simulink model "b0307"  (R2025b)
settings: Solver=ode4  StartTime=0.0  StopTime=533  FixedStep=0.001  RelTol=1e-3
values from neighbouring files (symbols this model uses):
  alpha_vector = [-8 -4 -2 0 2 3 4 5 6 8 10 12]    [aerodata.mat]    (also in airdate.m = [-8 -4 -2 0 2 3 4 5 6 8 10 12]')
  alpha_vector1 = [-4 0 4 8]    [aerodata.mat]    (also in airdate.m = [-4, 0, 4, 8])
  alpha_vector2 = [-4 0 4 8]    [aerodata.mat]    (also in airdate.m = [-4, 0, 4, 8])
  b_ref = 2.24    [init.m]
  beta_vector1 = [-8 -4 0 4 8]    [aerodata.mat]    (also in airdate.m = [-8, -4, 0, 4, 8])
  c_ref = 0.165    [init.m]
  CD_alpha = [0.0485620740363 0.0318356514345 0.0317790643102 0.0364045204537 0.0445214008185 0.0513240541996 0.0580305477533 0.0657045426134 0.0744839493029 0.0955551011208 0.133141813384 0.18014601666]    [aerodata.mat]    (also in airdate.m = alpha_matrix(1:length(alpha_vector), 3))
  CD_beta = [0.0413061898506 0.0345389961433 0.0318356514345 0.0345389961433 0.0413061898506 0.0436826 0.0385768 0.0364045204537 0.0371657170379 0.0408604078007 0.0616785 0.0590205 ... (20 elements, 5x4)]    [aerodata.mat]    (also in airdate.m = reshape(beta_matrix(:, 3), [n_beta, n_alpha1]))
  CD_ELE = [0.0367807192259 0.0308673912055 0.0306770192219 0.0329799710874 0.0376266798938 0.0362372767671 0.0347486720958 0.0364045204537 0.0395900797854 0.0493584368547 0.0520155680915 0.0546030505455 ... (20 elements, 5x4)]    [aerodata.mat]    (also in airdate.m = reshape(def_ELE_L_matrix(:, 4), [n_ele, n_alpha2]))
  CL_alpha = [-0.316928256932 -0.0246785813034 0.130283368141 0.288945629191 0.449323999783 0.525648685194 0.60297649153 0.678148219772 0.750129216407 0.872962476804 0.920788454091 0.929116005788]    [aerodata.mat]    (also in airdate.m = alpha_matrix(1:length(alpha_vector), 5))
  Cl_alpha = [-0.000640872979326 1.08116418077e-05 2.92649499784e-07 0 -0.000437066219056 -0.000762440123061 -0.000973039479867 -0.00125684277681 -0.00152984821199 -0.00187186802219 -0.00184918573213 0.00105936824418]    [aerodata.mat]    (also in airdate.m = alpha_matrix(1:length(alpha_vector), 6))
  CL_beta = [-0.0254603323809 -0.0249297140554 -0.0246785813034 -0.0249297140554 -0.0254603323809 0.27807 0.286078 0.288945629191 0.286671909097 0.27925707766 0.602944 0.604359 ... (20 elements, 5x4)]    [aerodata.mat]    (also in airdate.m = reshape(beta_matrix(:, 5), [n_beta, n_alpha1]))
  Cl_beta = [0.000236297001567 0.000139283426539 1.08116418077e-05 -0.000139283426539 -0.000236297001567 0.000738099 0.000299952 -0.000269027677603 -0.00096883985561 -0.00179948469019 0.0018278 0.000411742 ... (20 elements, 5x4)]    [aerodata.mat]    (also in airdate.m = reshape(beta_matrix(:, 6), [n_beta, n_alpha1]))
  CL_ELE = [-0.209245674304 -0.118097376915 -0.0691301102129 -0.0258480382303 0.0604619193477 0.145712419951 0.241076881119 0.288945629191 0.337037782187 0.427489906586 0.461138992576 0.556875751161 ... (20 elements, 5x4)]    [aerodata.mat]    (also in airdate.m = reshape(def_ELE_L_matrix(:, 6), [n_ele, n_alpha2]))
  Cl_ELE = [-0.0251269797289 -0.008426817179 0.000240167384607 0.00909972758991 0.0243415498089 -0.0265884432031 -0.00914521718395 -0.000269027677603 0.00845228310052 0.0248325485851 -0.027436226674 -0.00980497383292 ... (20 elements, 5x4)]    [aerodata.mat]    (also in airdate.m = reshape(def_ELE_L_matrix(:, 7), [n_ele, n_alpha2]))
  Cl_ELER = [0.0251269797289 0.008426817179 -0.000240167384607 -0.00909972758991 -0.0243415498089 0.0265884432031 0.00914521718395 0.000269027677603 -0.00845228310052 -0.0248325485851 0.027436226674 0.00980497383292 ... (20 elements, 5x4)]    [aerodata.mat]    (also in airdate.m = -Cl_ELE)
  Cm_alpha = [0.0626600725128 0.0530799370217 0.0636683163616 0.0662391704182 0.0712518097577 0.059404297375 0.0463976401398 0.0265816846325 -0.000744425674427 -0.0975303788137 -0.390110677431 -0.549514574144]    [aerodata.mat]    (also in airdate.m = alpha_matrix(1:length(alpha_vector), 7))
  Cm_beta = [0.0443576401398 0.0504624 0.0530799370217 0.0504624 0.0443576401398 0.0399653 0.0540624 0.0662391704182 0.0664956832735 0.054831924477 -0.0180401 0.0135503 ... (20 elements, 5x4)]    [aerodata.mat]    (also in airdate.m = reshape(beta_matrix(:, 7), [n_beta, n_alpha1]))
  Cm_ELE = [0.536255917663 0.147824254744 -0.0380057879786 -0.216266528425 -0.571251073338 0.641418774301 0.260817426469 0.0662391704182 -0.124486673615 -0.489660800762 0.614897515281 0.238355554417 ... (20 elements, 5x4)]    [aerodata.mat]    (also in airdate.m = reshape(def_ELE_L_matrix(:, 8), [n_ele, n_alpha2]))
  Cn_alpha = [-0.000921303455433 -0.000100429360075 -5.32721662229e-05 0 -0.000448050865233 -0.000265660085507 -0.000172455805371 -9.0297395806e-05 0.000114919609077 0.000960640598216 0.000800025371357 0.00296984280205]    [aerodata.mat]    (also in airdate.m = alpha_matrix(1:length(alpha_vector), 8))
  Cn_beta = [-0.0118929295373 -0.00644657732457 -0.000100429360075 0.00644657732457 0.0118929295373 -0.00932594 -0.00455936 -0.000185600362027 0.00379534502079 0.00738347341913 -0.00140779 -0.00161764 ... (20 elements, 5x4)]    [aerodata.mat]    (also in airdate.m = reshape(beta_matrix(:, 8), [n_beta, n_alpha1]))
  Cn_ELE = [-0.000978013358228 0.000374192483935 0.000921206928251 0.00041612460588 -0.00121710528947 -0.00219374024917 -0.000325070715732 -0.000185600362027 -8.6022941264e-05 -0.000494144283219 -0.00293821245405 -0.00054824676514 ... (20 elements, 5x4)]    [aerodata.mat]    (also in airdate.m = reshape(def_ELE_L_matrix(:, 9), [n_ele, n_alpha2]))
  Cn_ELER = [0.000978013358228 -0.000374192483935 -0.000921206928251 -0.00041612460588 0.00121710528947 0.00219374024917 0.000325070715732 0.000185600362027 8.6022941264e-05 0.000494144283219 0.00293821245405 0.00054824676514 ... (20 elements, 5x4)]    [aerodata.mat]    (also in airdate.m = -Cn_ELE)
  CY_alpha = [0.00094331940582 8.91316440807e-05 0.00163191368255 0 0.00399491029065 0.00495876756067 0.00538171092978 0.00589122371949 0.00623993707833 0.00649420059364 0.0115896523304 0.0134657730505]    [aerodata.mat]    (also in airdate.m = alpha_matrix(1:length(alpha_vector), 4))
  CY_beta = [0.0411779977966 0.0260529022214 8.91316440807e-05 -0.0260529022214 -0.0411779977966 0.0626258 0.0323129 0.00352355870293 -0.0237421290295 -0.0494841840717 0.0422501 0.0258494 ... (20 elements, 5x4)]    [aerodata.mat]    (also in airdate.m = reshape(beta_matrix(:, 4), [n_beta, n_alpha1]))
  CY_ELE = [0.00947355235179 0.0032440045221 0.000919743913066 3.31170671791e-05 -0.00246607912146 0.00984559930618 0.00470476147172 0.00352355870293 0.00144187166173 -0.00241087659802 0.0116316527742 0.00697261934365 ... (20 elements, 5x4)]    [aerodata.mat]    (also in airdate.m = reshape(def_ELE_L_matrix(:, 5), [n_ele, n_alpha2]))
  def_ELE_L_vector = [-15 -5 0 5 15]    [aerodata.mat]    (also in airdate.m = [-15, -5, 0, 5, 15])
  delta_max = 15    [init.m]
  fly_pt = [0 397.202504295 825.49541327 510 4564.45331975 4885.85117615 4860 4885.85117615 4899.67498335 5610.29789652 5624.12170371 5880 ... (135 elements, 27x5)]    [baseline_fly_plan.mat]    (also in debug_replay_flyphase.m = evalin('base','fly_pt'); dubins_path_planning.m = dubins.filter_waypoints(fly_pt); fly_planfjy.mat; make_orbit_plan.m = dubins.filter_waypoints(fly_pt))
  g = 9.8    [Astar.m]    (also in dubins_path_planning.m; init.m; make_orbit_plan.m; make_route_plan.m)
  I = [I_x -I_xy -I_xz ... (first row only)    [init.m]
  I_inv = inv(I)    [init.m]
  kal = (wn^2-a_24(3))/(2*zeta*wn)    [controller.m]
  ki = 0.1*kphi    (= 0.75)    [controller.m]
  kn = (-2.2*wn^2*g)/(Tr*(wn^2+a_24(3))*Vc*Z_al)    [controller.m]
  kp = 2*zeta2*wn2/N_delatr_bar    [controller.m]
  kphi = wn2/2/zeta2    (= 7.5)    [controller.m]
  kq = -(2*zeta*wn) / a_25    [controller.m]
  mass = 27.1    [init.m]
  pitch_max = 30    [init.m]
  psi_0 = 0 * (pi/180)    (= 0)    [init.m]
  psi_t = 0    [Astar.m]    (also in init.m)
  roll_max = 30*pi/180    (= 0.523598775598)    [Astar.m]    (also in dubins_path_planning.m = 0.261799387799; init.m = 30)
  S_ref = 0.7    [init.m]
  theta_0 = 30 * (pi/180)    (= 0.523598775598)    [init.m]
  theta_t = 0    [Astar.m]    (also in init.m)
  u_0 = Vc_0*cos(beta_0)*cos(alpha_0)    [init.m]
  v_0 = Vc_0*sin(beta_0)    [init.m]
  V_t = 0    [Astar.m]    (also in init.m)
  Vc = 34    [Astar.m]    (also in dubins_path_planning.m; init.m; make_orbit_plan.m; make_route_plan.m)
  w_0 = Vc_0*cos(beta_0)*sin(alpha_0)    [init.m]
  W_down = 0    [init.m]
  W_east = 0    [init.m]
  W_north = 0    [init.m]
  xt0 = 6500    [Astar.m]    (also in init.m)
  yt0 = 9000    [Astar.m]    (also in init.m)
  Z_al = (CD_alpha(10)+CL_al)*(q_0*S_ref/(mass*Vc))    [controller.m]
  zt0 = 0    [Astar.m]    (also in init.m)
undefined symbols (not defined in the file or in its folder): beta_vector0
libraries: matrix_library x2, simulink x1, aerolibatmos2 x1, slpidlib x1
(part 1 of 2)
settings Model: SimulationMode=accelerator  Creator=fjy  LastModifiedBy=fjy
settings SolverCC: ZeroCrossAlgorithm=Adaptive
settings DebuggingCC: IgnoredZcDiagnostic=none

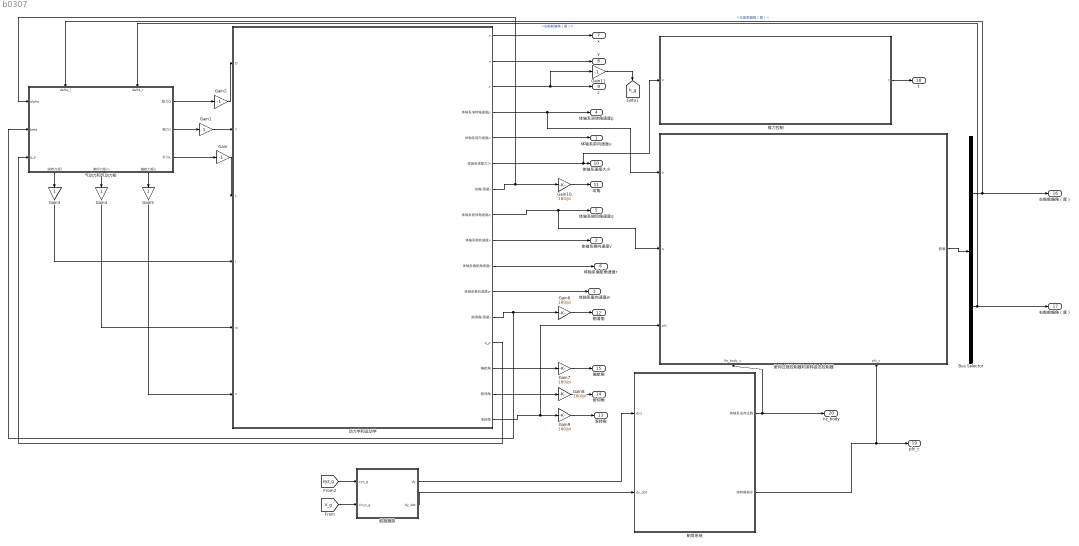
== system b0307 ==
  Bus Selector : BusSelector  OutputSignals=左舵舵偏角（度）,右舵舵偏角（度）
  Gain : Gain  Gain=-1
  Gain{1,3..5} (4 alike) : Gain
  Gain{6..10} (5 alike) : Gain  Gain=180/pi
  Gain11 : Gain  Gain=-1
  Gain2 : Gain  Gain=-1
  俯仰过载控制器和滚转姿态控制器 : Subsystem
      settings: PortSchema="{\"entries\":[{\"content\":{\"sides\":[{\"content\":{\"connectorIds\":[\"In1\",\"In2\",\"In3\"]},\"type\":\"ConnectorPlacement.EquallySpacedRectSide\",\"uuid\":\"d91e961c-baf5-4886-a4c8-008de2fd6bee\"},{\"content\":{\"connectorIds\":[\"Out1\"],\"side\":\"RIGHT\"},\"type\":\"ConnectorPlacement.EquallySpacedRectSide\",\"uuid\":\"2f89049f-57ed-40e6-8a3b-41aca5386f18\"},{\"content\":{\"side\":\"TOP\"},\"type\":\"ConnectorPlacement.EquallySpacedRectSide\",\"uuid\":\"4b65b47e-b030-4938-acd8-ff59fd67c9ad\"},{\"content\":{\"connectorIds\":[\"In4\",\"In5\"],\"side\":\"BOTTOM\"},\"type\":\"ConnectorPlacement.EquallySpacedRectSide\",\"uuid\":\"81f4b276-44af-4660-9fd9-5cca4e185003\"}]},\"type\":\"ConnectorPlacement.EquallySpacedConnector\",\"uuid\":\"4d45e1fc-459f-4755-b3f8-d77370a73e9c\"}],\"packageUris\":[\"http://schema.mathworks.com/mf0/Connector/R2020b\"],\"version\":\"1.0\"}"
  制导系统 : Subsystem
  动力学和运动学 : Subsystem
  推力控制 : Subsystem
  气动力和气动力矩 : Subsystem
      settings: PortSchema="{\"entries\":[{\"content\":{\"sides\":[{\"content\":{\"connectorIds\":[\"In1\",\"In2\",\"In3\"]},\"type\":\"ConnectorPlacement.EquallySpacedRectSide\",\"uuid\":\"0d84a32f-2cac-4fa1-9193-2f4fbb725518\"},{\"content\":{\"connectorIds\":[\"Out1\",\"Out2\",\"Out3\"],\"side\":\"RIGHT\"},\"type\":\"ConnectorPlacement.EquallySpacedRectSide\",\"uuid\":\"18d8cbb4-08a2-4061-89fa-8dc7627fca90\"},{\"content\":{\"connectorIds\":[\"In4\",\"In5\"],\"side\":\"TOP\"},\"type\":\"ConnectorPlacement.EquallySpacedRectSide\",\"uuid\":\"86ac52b9-0ecc-4c2f-bfe2-1b5376181286\"},{\"content\":{\"connectorIds\":[\"Out4\",\"Out5\",\"Out6\"],\"side\":\"BOTTOM\"},\"type\":\"ConnectorPlacement.EquallySpacedRectSide\",\"uuid\":\"b98cec75-1790-4cd7-b7eb-ef9c637c8472\"}]},\"type\":\"ConnectorPlacement.EquallySpacedConnector\",\"uuid\":\"ecac8566-2709-47ed-83ad-8cea7f87013b\"}],\"packageUris\":[\"http://schema.mathworks.com/mf0/Connector/R2020b\"],\"version\":\"1.0\"}"
  航路跟踪 : Subsystem
  体轴系前向速度u : Outport
  体轴系侧向速度v : Outport  Port=2
  体轴系垂向速度w : Outport  Port=3
  体轴系滚转角速度p : Outport  Port=4
  体轴系俯仰角速度q : Outport  Port=5
  体轴系偏航角速度r : Outport  Port=6
  x : Outport  Port=7
  y : Outport  Port=8
  z : Outport  Port=9
  体轴系速度大小 : Outport  Port=10
  攻角 : Outport  Port=11
  侧滑角 : Outport  Port=12
  滚转角 : Outport  Port=13
  俯仰角 : Outport  Port=14
  偏航角 : Outport  Port=15
  左舵舵偏角（度） : Outport  Port=16
  右舵舵偏角（度） : Outport  Port=17
  t : Outport  Port=18
  phi_c : Outport  Port=19
  nz_body : Outport  Port=20
  tag scope: h_g=global
  wires:
  动力学和运动学/13(q_p) -> 气动力和气动力矩/3(q_p)
  气动力和气动力矩/3(升力L) -> Gain/1
  气动力和气动力矩/1(阻力D) -> Gain2/1
  气动力和气动力矩/2(侧力Y) -> Gain1/1
  气动力和气动力矩/4(滚转力矩l) -> Gain3/1
  气动力和气动力矩/5(俯仰力矩m) -> Gain4/1
  气动力和气动力矩/6(偏航力矩n) -> Gain5/1
  Gain2/1 -> 动力学和运动学/1(D)
  Gain1/1 -> 动力学和运动学/2(Y)
  Gain/1 -> 动力学和运动学/3(L)
  Gain3/1 -> 动力学和运动学/4(l)
  Gain4/1 -> 动力学和运动学/5(m)
  Gain5/1 -> 动力学和运动学/6(n)
  动力学和运动学/1(x) -> x/1
  动力学和运动学/2(y) -> y/1
  动力学和运动学/3(z) -> Gain11/1, z/1
  动力学和运动学/4(体轴系滚转角速度p) -> 俯仰过载控制器和滚转姿态控制器/1(p), 体轴系滚转角速度p/1
  动力学和运动学/5(体轴系前向速度u) -> 体轴系前向速度u/1
  动力学和运动学/6(体轴系速度大小) -> 推力控制/1(V), 体轴系速度大小/1
  动力学和运动学/8(体轴系俯仰角速度q) -> 俯仰过载控制器和滚转姿态控制器/2(q), 体轴系俯仰角速度q/1
  动力学和运动学/9(体轴系侧向速度v) -> 体轴系侧向速度v/1
  动力学和运动学/10(体轴系偏航角速度r) -> 体轴系偏航角速度r/1
  动力学和运动学/11(体轴系垂向速度w) -> 体轴系垂向速度w/1
  动力学和运动学/7(攻角(弧度)) -> 气动力和气动力矩/1(alpha), Gain10/1
  动力学和运动学/12(侧滑角(弧度)) -> Gain6/1, 气动力和气动力矩/2(beta)
  动力学和运动学/16(滚转角) -> 俯仰过载控制器和滚转姿态控制器/3(phi), Gain9/1
  动力学和运动学/14(偏航角) -> Gain7/1
  Gain6/1 -> 侧滑角/1
  Gain7/1 -> 偏航角/1
  Gain8/1 -> 俯仰角/1
  Gain9/1 -> 滚转角/1
  Gain10/1 -> 攻角/1
  Bus Selector/2 -> 右舵舵偏角（度）/1, 气动力和气动力矩/5(delta_r)  "<右舵舵偏角（度）>"
  Bus Selector/1 -> 左舵舵偏角（度）/1, 气动力和气动力矩/4(delta_l)  "<左舵舵偏角（度）>"
  推力控制/1(t) -> t/1
  俯仰过载控制器和滚转姿态控制器/1(舵偏) -> Bus Selector/1
  Gain11/1 -> [h_g]
  动力学和运动学/15(俯仰角) -> Gain8/1
  制导系统/1(体轴系法向过载) -> nz_body/1, 俯仰过载控制器和滚转姿态控制器/4(Nz_body_c)
  制导系统/2(滚转角指令) -> 俯仰过载控制器和滚转姿态控制器/5(phi_c), phi_c/1
  [xyz_g] -> 航路跟踪/1(xyz_g)
  [V_g] -> 航路跟踪/2(Vxyz_g)
  航路跟踪/2(dy_dot) -> 制导系统/2(dy_dot)
  航路跟踪/1(dy) -> 制导系统/1(dy1)

== system b0307/俯仰过载控制器和滚转姿态控制器 ==
  p : Inport
  q : Inport  Port=2
  phi : Inport  Port=3
  Nz_body_c : Inport  Port=4
  phi_c : Inport  Port=5
  俯仰过载控制器 : Subsystem
  滚转姿态控制器 : Subsystem
  舵分配 : Subsystem
  Out Bus Element : Outport  PortName=舵偏  Element=左舵舵偏角（度）
  Out Bus Element1 : Outport  PortName=舵偏  Element=右舵舵偏角（度）
  wires:
  q/1 -> 俯仰过载控制器/1(q)
  phi/1 -> 滚转姿态控制器/3(phi)
  p/1 -> 滚转姿态控制器/1(p)
  俯仰过载控制器/1(俯仰控制舵偏角（度）) -> 舵分配/1(俯仰控制舵偏角（度）)
  滚转姿态控制器/1(滚转控制舵偏角（度）) -> 舵分配/2(滚转控制舵偏角（度）)
  Nz_body_c/1 -> 俯仰过载控制器/2(Nz_body_c)
  phi_c/1 -> 滚转姿态控制器/2(phi_c)
  舵分配/2(右舵舵偏角（度）) -> Out Bus Element1/1
  舵分配/1(左舵舵偏角（度）) -> Out Bus Element/1

== system b0307/制导系统 ==
  dy1 : Inport
  dy_dot : Inport  Port=2
  制导系统 : Subsystem
  相对运动学模型 : Subsystem
  体轴系法向过载 : Outport
  滚转角指令 : Outport  Port=2
  wires:
  相对运动学模型/3(视线方位角速率（弧度）) -> 制导系统/5(视线方位角速率)
  [V_g] -> 相对运动学模型/2(飞行器地面系速度)
  相对运动学模型/2(视线高低角速率(弧度)) -> 制导系统/4(视线高低角速率)
  [xyz_g] -> 相对运动学模型/1(飞行器地面系位置)
  相对运动学模型/1(俯仰角（弧度）) -> 制导系统/3(俯仰角(弧度))
  制导系统/2(滚转角指令) -> 滚转角指令/1
  制导系统/1(体轴系法向过载) -> 体轴系法向过载/1
  dy1/1 -> 制导系统/1(dy1)
  dy_dot/1 -> 制导系统/2(dy_dot)
  相对运动学模型/4(视线高低角) -> 制导系统/6(视线高低角)

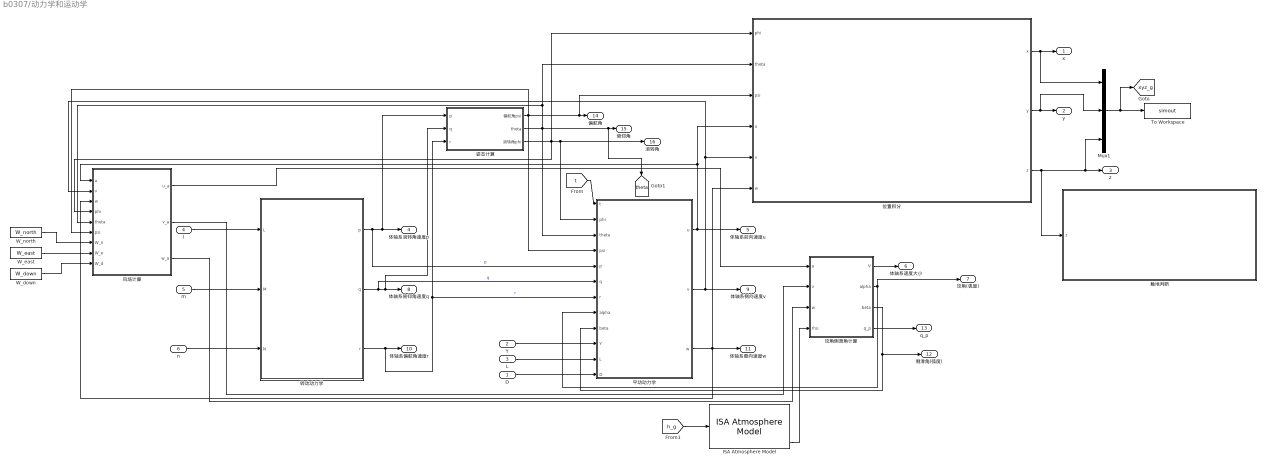
== system b0307/动力学和运动学 ==
  D : Inport
  Y : Inport  Port=2
  L : Inport  Port=3
  l : Inport  Port=4
  m : Inport  Port=5
  n : Inport  Port=6
  ISA Atmosphere Model : aerolibatmos2/ISA Atmosphere Model  useExtended=off  action=None  custom=off  viscosityOut=off  g=9.80665  gamma=1.4  R=287.0531  L=0.0065  h_trop=11000  h_strat=20000  rho0=1.225  P0=101325  T0=288.15  h0=0  S=110.4  Tref=273.15  muref=1.716e-5
  Mux1 : Mux  Inputs=3
  To Workspace : ToWorkspace  VariableName=simout  SaveFormat=Timeseries  SampleTime=-1
  W_down : Constant  Value=W_down
  W_east : Constant  Value=W_east
  W_north : Constant  Value=W_north
  位置积分 : Subsystem
  姿态计算 : Subsystem
  平动动力学 : Subsystem
  攻角侧滑角计算 : MATLAB Function  TreatAsAtomicUnit=on
  触地判断 : Subsystem
  转动动力学 : Subsystem
  风场计算 : MATLAB Function  TreatAsAtomicUnit=on
  x : Outport
  y : Outport  Port=2
  z : Outport  Port=3
  体轴系滚转角速度p : Outport  Port=4
  体轴系前向速度u : Outport  Port=5
  体轴系速度大小 : Outport  Port=6
  攻角(弧度) : Outport  Port=7
  体轴系俯仰角速度q : Outport  Port=8
  体轴系侧向速度v : Outport  Port=9
  体轴系偏航角速度r : Outport  Port=10
  体轴系垂向速度w : Outport  Port=11
  侧滑角(弧度) : Outport  Port=12
  q_p : Outport  Port=13
  偏航角 : Outport  Port=14
  俯仰角 : Outport  Port=15
  滚转角 : Outport  Port=16
  tag scope: theta=global, xyz_g=global
  wires:
  Mux1/1 -> To Workspace/1, [xyz_g]
  转动动力学/1(p) -> 体轴系滚转角速度p/1, 姿态计算/1(p), 平动动力学/5(p)  "p"
  攻角侧滑角计算/2(alpha) -> 攻角(弧度)/1, 平动动力学/8(alpha)
  攻角侧滑角计算/3(beta) -> 平动动力学/9(beta), 侧滑角(弧度)/1
  姿态计算/3(滚转角phi) -> 风场计算/4(phi), 位置积分/1(phi), 平动动力学/2(phi), 滚转角/1
  平动动力学/1(u) -> 风场计算/1(u), 位置积分/4(u), 体轴系前向速度u/1
  平动动力学/3(w) -> 风场计算/3(w), 位置积分/6(w), 体轴系垂向速度w/1
  D/1 -> 平动动力学/12(D)
  ISA Atmosphere Model/4 -> 攻角侧滑角计算/4(rho)
  转动动力学/3(r) -> 体轴系偏航角速度r/1, 姿态计算/3(r), 平动动力学/7(r)  "r"
  攻角侧滑角计算/4(q_p) -> q_p/1
  位置积分/1(x) -> x/1, Mux1/1
  平动动力学/2(v) -> 风场计算/2(v), 位置积分/5(v), 体轴系侧向速度v/1
  L/1 -> 平动动力学/11(L)
  转动动力学/2(q) -> 体轴系俯仰角速度q/1, 姿态计算/2(q), 平动动力学/6(q)  "q"
  攻角侧滑角计算/1(V) -> 体轴系速度大小/1
  Y/1 -> 平动动力学/10(Y)
  [t] -> 平动动力学/1(t)
  位置积分/2(y) -> y/1, Mux1/2
  姿态计算/1(偏航角psi) -> 风场计算/6(psi), 平动动力学/4(psi), 位置积分/3(psi), 偏航角/1
  n/1 -> 转动动力学/3(N)
  l/1 -> 转动动力学/1(L)
  m/1 -> 转动动力学/2(M)
  位置积分/3(z) -> 触地判断/1(z), z/1, Mux1/3
  [h_g] -> ISA Atmosphere Model/1
  姿态计算/2(theta) -> 风场计算/5(theta), 位置积分/2(theta), 平动动力学/3(theta), [theta], 俯仰角/1
  风场计算/1(u_a) -> 攻角侧滑角计算/1(u)
  风场计算/2(v_a) -> 攻角侧滑角计算/2(v)
  风场计算/3(w_a) -> 攻角侧滑角计算/3(w)
  W_north/1 -> 风场计算/7(W_n)
  W_east/1 -> 风场计算/8(W_e)
  W_down/1 -> 风场计算/9(W_d)

== system b0307/推力控制 ==
  V : Inport
  Constant : Constant  Value=Vc
  Constant1 : Constant  Value=200
  Gain : Gain
  PID Controller2 : slpidlib/PID Controller  Controller=PID  Form=Parallel  TimeDomain=Continuous-time  UseExternalTs=off  SampleTime=-1  IntegratorMethod=Forward Euler  FilterMethod=Forward Euler  ControllerParametersSource=internal  P=3  I=1  UseKiTs=off  D=0  UseExternalDerivativeSource=off  N=0  UseFilter=on  TunerSelectOption=Transfer Function Based (PID Tuner App)  InitialConditionSource=internal  InitialConditionForIntegrator=0  InitialConditionForFilter=0  DifferentiatorICPrevScaledInput=0  ExternalReset=none  TrackingMode=off  Kt=1  LimitOutput=on  SatLimitsSource=internal  UpperSaturationLimit=1  LowerSaturationLimit=0  LinearizeAsGain=on  AntiWindupMode=clamping  Kb=1  LimitIntegrator=off  UpperIntegratorSaturationLimit=inf  LowerIntegratorSaturationLimit=-inf  POutMin=[]  POutMax=[]  IOutMin=[]  IOutMax=[]  DOutMin=[]  DOutMax=[]  NOutMin=[]  NOutMax=[]  SumOutMin=[]  SumOutMax=[]  SaturationOutMin=[]  SaturationOutMax=[]  PParamMin=[]  PParamMax=[]  IParamMin=[]  IParamMax=[]  DParamMin=[]  DParamMax=[]  NParamMin=[]  NParamMax=[]  KbParamMin=[]  KbParamMax=[]  KtParamMin=[]  KtParamMax=[]  KbOutMin=[]  KbOutMax=[]  KtOutMin=[]  KtOutMax=[]  IntegratorOutMin=[]  IntegratorOutMax=[]  FilterOutMin=[]  FilterOutMax=[]  SumI1OutMin=[]  SumI1OutMax=[]  SumI2OutMin=[]  SumI2OutMax=[]  SumI3OutMin=[]  SumI3OutMax=[]  SumI4OutMin=[]  SumI4OutMax=[]  SumDOutMin=[]  SumDOutMax=[]  DifferentiatorOutMin=[]  DifferentiatorOutMax=[]  FilterDiffOutCoefMin=[]  FilterDiffOutCoefMax=[]  ReciprocalOutMin=[]  ReciprocalOutMax=[]  SumDenOutMin=[]  SumDenOutMax=[]  SumNumOutMin=[]  SumNumOutMax=[]  DivideOutMin=[]  DivideOutMax=[]  UdiffTsProdOutMin=[]  UdiffTsProdOutMax=[]  NTsProdOutMin=[]  NTsProdOutMax=[]  UintegralTsProdOutMin=[]  UintegralTsProdOutMax=[]  UngainTsProdOutMin=[]  UngainTsProdOutMax=[]  ClampingZeroOutDataTypeStr=Inherit: Inherit via back propagation  ClampingZeroOutMin=[]  ClampingZeroOutMax=[]  FilterDenConstantOutDataTypeStr=Inherit: Inherit via back propagation  FilterDenConstantOutMin=[]  FilterDenConstantOutMax=[]  PCopyOutDataTypeStr=Inherit: Inherit via back propagation  PCopyOutMin=[]  PCopyOutMax=[]  NCopyOutDataTypeStr=Inherit: Inherit via back propagation  NCopyOutMin=[]  NCopyOutMax=[]  IntegratorContinuousStateAttributes=''  IntegratorStateMustResolveToSignalObject=off  IntegratorRTWStateStorageClass=Auto  FilterContinuousStateAttributes=''  FilterStateMustResolveToSignalObject=off  FilterRTWStateStorageClass=Auto  ParallelPVariant=InternalParameters  IdealPVariant=Disabled  IVariant=InternalParameters  DVariant=InternalParameters  IntegratorVariant=Continuous  SatVariant=Enabled  AWVariant=ContClampingParallel  PCopyVariant=Disabled  TRVariant=Disabled  FdbkBlocksVariant=Forward  IdealPFdbkVariant=Disabled  SatFdbkVariant=Disabled  DerivativeFilterVariant=ContFilter  NVariant=InternalParameters  NCopyVariant=Disabled  FilterICVariant=InternalICsFilter  IntegratorICVariant=InternalICs  ExternalResetVariant=Disabled  TRSumVariant=Passthrough  SumFdbkVariant=Disabled  SumVariant=Sum_PID  TsampFilterVariant=InternalTs  TsampNgainVariant=Passthrough  TsampIntegralVariant=Disabled_SignalSpec  ExternalSaturationOutDataTypeStr=Inherit: Same as second input  DerivativeSourceVariant=ErrorSignal  PreIntVariant=InternalPreInt
  Product : Product
  Sum : Sum  Inputs=|+-
  To Workspace : ToWorkspace  VariableName=thrust_cmd  SaveFormat=Timeseries  SampleTime=-1
  t : Outport
  tag scope: t=global
  wires:
  Constant1/1 -> Product/1
  Product/1 -> To Workspace/1, t/1, [t]
  V/1 -> Sum/2
  PID Controller2/1 -> Gain/1
  Constant/1 -> Sum/1
  Sum/1 -> PID Controller2/1
  Gain/1 -> Product/2

== system b0307/气动力和气动力矩 ==
  alpha : Inport
  beta : Inport  Port=2
  q_p : Inport  Port=3
  delta_l : Inport  Port=4
  delta_r : Inport  Port=5
  Gain : Gain  Gain=180/3.14
  Gain1 : Gain  Gain=180/3.14
  Gain2 : Gain
  Gain3 : Gain
  Gain4 : Gain
  Saturation : Saturate  UpperLimit=12  LowerLimit=-8
  Saturation1 : Saturate  UpperLimit=8  LowerLimit=-8
  气动力 : Subsystem
  气动力矩 : Subsystem
  阻力D : Outport
  侧力Y : Outport  Port=2
  升力L : Outport  Port=3
  滚转力矩l : Outport  Port=4
  俯仰力矩m : Outport  Port=5
  偏航力矩n : Outport  Port=6
  wires:
  alpha/1 -> Gain1/1
  q_p/1 -> 气动力矩/1(q_p), 气动力/1(q_p)
  气动力/3(升力L) -> 升力L/1
  气动力/1(阻力D) -> 阻力D/1
  Saturation/1 -> 气动力矩/3(alpha), 气动力/3(alpha)
  beta/1 -> Gain/1
  Saturation1/1 -> 气动力矩/2(beta), 气动力/2(beta)
  气动力/2(侧力Y) -> Gain4/1
  气动力矩/1(滚转力矩l) -> Gain2/1
  气动力矩/3(偏航力矩n) -> Gain3/1
  气动力矩/2(俯仰力矩m) -> 俯仰力矩m/1
  Gain/1 -> Saturation1/1
  Gain1/1 -> Saturation/1
  delta_l/1 -> 气动力矩/4(delta_l), 气动力/4(delta_l)
  delta_r/1 -> 气动力矩/5(delta_r), 气动力/5(delta_r)
  Gain2/1 -> 滚转力矩l/1
  Gain3/1 -> 偏航力矩n/1
  Gain4/1 -> 侧力Y/1

== system b0307/航路跟踪 ==
  xyz_g : Inport
  Vxyz_g : Inport  Port=2
  Clock : Clock
  Constant : Constant  Value=fly_pt
  Display : Display
  MATLAB Function : MATLAB Function  TreatAsAtomicUnit=on
  MATLAB Function1 : MATLAB Function  TreatAsAtomicUnit=on
  Scope{1..4} (4 alike) : Scope
      Scope1 settings: ActiveDisplayYMinimum=-742.15143659092359  ActiveDisplayYMaximum=6679.4046232625515  DataLoggingVariableName=ScopeData6
      Scope2 settings: ActiveDisplayYMinimum=-1.3749999999999996  ActiveDisplayYMaximum=22.375  DataLoggingVariableName=ScopeData2
      Scope3 settings: ActiveDisplayYMinimum=-11.237909512986135  ActiveDisplayYMaximum=15.91784653976285  DataLoggingVariableName=ScopeData25
      Scope4 settings: ActiveDisplayYMinimum=-72.782202892880449  ActiveDisplayYMaximum=65.504144118786328  DataLoggingVariableName=ScopeData26
  Unit Delay : UnitDelay  SampleTime=-1  HasFrameUpgradeWarning=on
  Unit Delay1 : UnitDelay  SampleTime=-1  HasFrameUpgradeWarning=on
  coc : Display
  next : Display
  prev : Display
  dy : Outport
  dy_dot : Outport  Port=2
  tag scope: coc_pt=global, fly_type=global, next_pt=global, prev_pt=global
  wires:
  Constant/1 -> MATLAB Function/4(fly_pt)
  Clock/1 -> MATLAB Function/3(time)
  MATLAB Function/4(next_pt) -> MATLAB Function1/3(next_pt), next/1, [next_pt]
  xyz_g/1 -> MATLAB Function/5(xyz_g), MATLAB Function1/5(xyz_g)
  Vxyz_g/1 -> MATLAB Function1/6(Vxyz_g)
  MATLAB Function/1(fly_phase) -> Display/1, Scope2/1
  MATLAB Function1/2(dy_dot) -> dy_dot/1, Scope3/1
  MATLAB Function1/1(dy) -> Scope4/1, dy/1, Unit Delay1/1
  MATLAB Function1/3(DTG) -> Unit Delay/1, Scope1/1
  Unit Delay/1 -> MATLAB Function/2(DTG)
  Unit Delay1/1 -> MATLAB Function/1(dy)
  MATLAB Function/2(fly_type) -> [fly_type], MATLAB Function1/1(fly_type)
  MATLAB Function/3(prev_pt) -> prev/1, MATLAB Function1/2(prev_pt), [prev_pt]
  MATLAB Function/5(coc_pt) -> [coc_pt], MATLAB Function1/4(coc_pt), coc/1

== system b0307/俯仰过载控制器和滚转姿态控制器/俯仰过载控制器 ==
  q : Inport
  Nz_body_c : Inport  Port=2
  Gain11 : Gain  Gain=kn
  Gain12 : Gain  Gain=kal
  Gain13 : Gain  Gain=kq*180/pi
  Integrator : Integrator
  Saturation : Saturate  UpperLimit=pitch_max  LowerLimit=-pitch_max
  Scope : Scope  NumInputPorts=2
      settings: ActiveDisplayYMinimum=-2.5258005439869597  ActiveDisplayYMaximum=0.98568844574071224  DataLoggingVariableName=ScopeData7
  Sum : Sum  Inputs=|+-
  Sum1 : Sum  Inputs=|+-
  Sum2 : Sum  Inputs=|+-
  To Workspace : ToWorkspace  VariableName=Nz_cmd  SaveFormat=Structure With Time  SampleTime=-1
  Transfer Fcn : TransferFcn  Denominator=[1 Z_al]
  计算过载 : Subsystem
  俯仰控制舵偏角（度） : Outport
  wires:
  Gain13/1 -> Saturation/1
  计算过载/1(nz) -> Scope/2, Sum/2
  Sum2/1 -> Gain13/1
  Sum1/1 -> Gain12/1
  Sum/1 -> Gain11/1
  Integrator/1 -> Sum1/1
  Gain11/1 -> Integrator/1
  Gain12/1 -> Sum2/1
  q/1 -> Transfer Fcn/1, Sum2/2
  Saturation/1 -> 俯仰控制舵偏角（度）/1
  Transfer Fcn/1 -> Sum1/2
  Nz_body_c/1 -> To Workspace/1, Scope/1, Sum/1

== system b0307/俯仰过载控制器和滚转姿态控制器/滚转姿态控制器 ==
  p : Inport
  phi_c : Inport  Port=2
  phi : Inport  Port=3
  Gain : Gain  Gain=pi/180
  Gain1 : Gain  Gain=180/pi
  Gain11 : Gain  Gain=kphi
  Gain13 : Gain  Gain=kp
  Gain2 : Gain  Gain=180/pi
  Gain4 : Gain  Gain=ki
  Integrator : Integrator
  Saturation : Saturate  UpperLimit=roll_max  LowerLimit=-roll_max
  Scope : Scope
      settings: ActiveDisplayYMinimum=-35.782161783540218  ActiveDisplayYMaximum=34.759556956888467
  Scope1 : Scope  NumInputPorts=2
      settings: ActiveDisplayYMinimum=-9.3554293305743936  ActiveDisplayYMaximum=13.719783196694262  DataLoggingVariableName=ScopeData8
  Sum : Sum  Inputs=|+-
  Sum1 : Sum  Inputs=|+-
  Sum2 : Sum  Inputs=|++
  滚转控制舵偏角（度） : Outport
  wires:
  Sum1/1 -> Gain13/1
  Saturation/1 -> 滚转控制舵偏角（度）/1
  p/1 -> Sum1/2
  phi/1 -> Gain2/1, Sum/2
  Integrator/1 -> Sum2/2
  Sum/1 -> Gain11/1, Gain4/1
  Gain4/1 -> Integrator/1
  Sum2/1 -> Sum1/1
  Gain11/1 -> Sum2/1
  Gain13/1 -> Gain1/1
  Gain1/1 -> Saturation/1
  Gain/1 -> Sum/1
  Gain2/1 -> Scope1/2
  phi_c/1 -> Scope1/1, Scope/1, Gain/1

== system b0307/俯仰过载控制器和滚转姿态控制器/舵分配 ==
  俯仰控制舵偏角（度） : Inport
  滚转控制舵偏角（度） : Inport  Port=2
  Abs : Abs  SaturateOnIntegerOverflow=off
  Abs1 : Abs  SaturateOnIntegerOverflow=off
  Add : Sum  Inputs=-+
  Constant : Constant  Value=pitch_max+roll_max
  MinMax : MinMax  Inputs=2
  Mux : Mux  Inputs=2
  Saturation : Saturate  UpperLimit=2*delta_max  LowerLimit=0
  Saturation1 : Saturate  UpperLimit=delta_max  LowerLimit=-delta_max
  Saturation2 : Saturate  UpperLimit=delta_max  LowerLimit=-delta_max
  Sign : Signum
  product : Product
  右舵 : Fcn  Expr=( -u[1] + u[2] ) / 2
  左舵 : Fcn  Expr=( u[1] + u[2] ) / 2
  左舵舵偏角（度） : Outport
  右舵舵偏角（度） : Outport  Port=2
  wires:
  Constant/1 -> Add/2
  Abs1/1 -> MinMax/2
  Add/1 -> Saturation/1
  俯仰控制舵偏角（度）/1 -> Sign/1, Abs1/1
  Abs/1 -> Add/1
  MinMax/1 -> product/1
  Saturation/1 -> MinMax/1
  Sign/1 -> product/2
  左舵/1 -> Saturation1/1
  右舵/1 -> Saturation2/1
  Mux/1 -> 右舵/1, 左舵/1
  Saturation1/1 -> 左舵舵偏角（度）/1
  Saturation2/1 -> 右舵舵偏角（度）/1
  product/1 -> Mux/2
  滚转控制舵偏角（度）/1 -> Mux/1, Abs/1

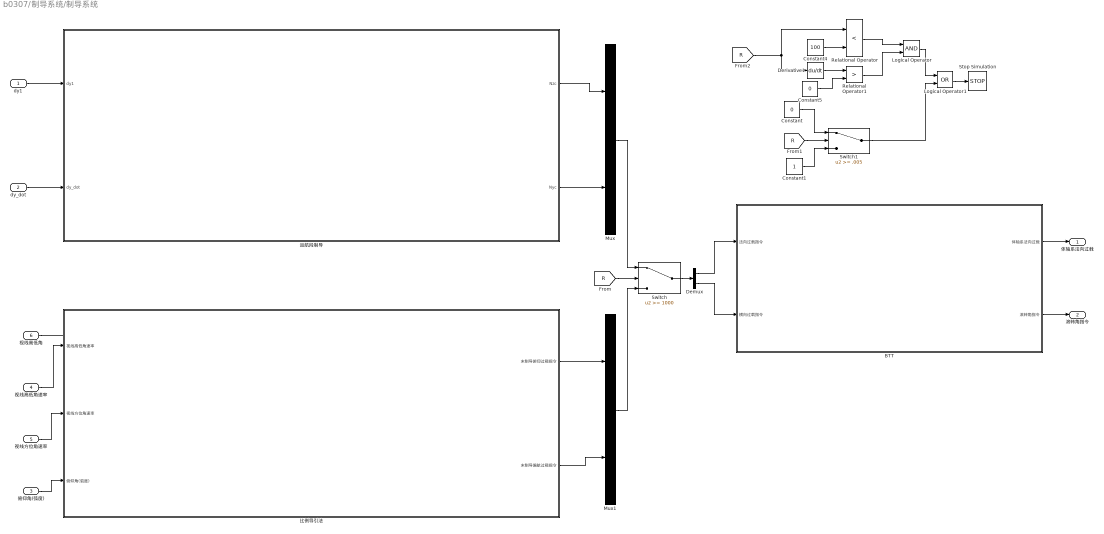
== system b0307/制导系统/制导系统 ==
  dy1 : Inport
  dy_dot : Inport  Port=2
  俯仰角(弧度) : Inport  Port=3
  视线高低角速率 : Inport  Port=4
  视线方位角速率 : Inport  Port=5
  视线高低角 : Inport  Port=6
  BTT : Subsystem
  Constant : Constant  Value=0
  Constant1 : Constant
  Constant4 : Constant  Value=100
  Constant5 : Constant  Value=0
  Demux : Demux  Outputs=2
  Derivative1 : Derivative
  Logical Operator : Logic  AllPortsSameDT=off  OutDataTypeStr=boolean
  Logical Operator1 : Logic  Operator=OR  AllPortsSameDT=off  OutDataTypeStr=boolean
  Mux : Mux  Inputs=2
  Mux1 : Mux  Inputs=2
  Relational Operator : RelationalOperator  Operator=<  OutDataTypeStr=boolean  RndMeth=Simplest  InputSameDT=off
  Relational Operator1 : RelationalOperator  Operator=>  OutDataTypeStr=boolean  RndMeth=Simplest  InputSameDT=off
  Stop Simulation : Stop
  Switch : Switch  Threshold=1000  SaturateOnIntegerOverflow=off  InputSameDT=off
  Switch1 : Switch  Threshold=.005  SaturateOnIntegerOverflow=off  InputSameDT=off
  巡航段制导 : Subsystem
  比例导引法 : Subsystem
  体轴系法向过载 : Outport
  滚转角指令 : Outport  Port=2
  wires:
  BTT/1(体轴系法向过载) -> 体轴系法向过载/1
  BTT/2(滚转角指令) -> 滚转角指令/1
  视线高低角速率/1 -> 比例导引法/1(视线高低角速率)
  视线方位角速率/1 -> 比例导引法/2(视线方位角速率)
  [R] -> Switch/2
  巡航段制导/1(Nzc) -> Mux/1
  巡航段制导/2(Nyc) -> Mux/2
  比例导引法/1(末制导俯仰过载指令) -> Mux1/1
  比例导引法/2(末制导偏航过载指令) -> Mux1/2
  Mux/1 -> Switch/1
  Mux1/1 -> Switch/3
  Demux/1 -> BTT/1(法向过载指令)
  Demux/2 -> BTT/2(横向过载指令)
  [R] -> Switch1/2
  Constant/1 -> Switch1/1
  Constant1/1 -> Switch1/3
  Switch/1 -> Demux/1
  俯仰角(弧度)/1 -> 比例导引法/3(俯仰角(弧度))
  dy1/1 -> 巡航段制导/1(dy1)
  dy_dot/1 -> 巡航段制导/2(dy_dot)
  Constant4/1 -> Relational Operator/2
  Relational Operator/1 -> Logical Operator/1
  Derivative1/1 -> Relational Operator1/1
  Constant5/1 -> Relational Operator1/2
  Relational Operator1/1 -> Logical Operator/2
  Logical Operator/1 -> Logical Operator1/1
  Switch1/1 -> Logical Operator1/2
  Logical Operator1/1 -> Stop Simulation/1
  [R] -> Derivative1/1, Relational Operator/1
  视线高低角/1 -> ?

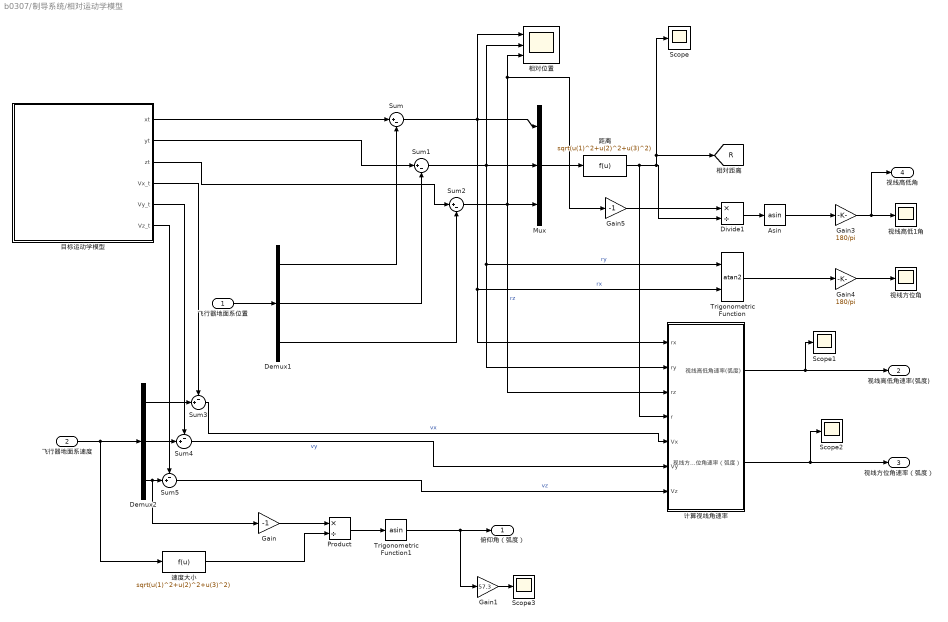
== system b0307/制导系统/相对运动学模型 ==
  飞行器地面系位置 : Inport
  飞行器地面系速度 : Inport  Port=2
  Asin : Trigonometry  Operator=asin
  Demux1 : Demux  Outputs=3
  Demux2 : Demux  Outputs=3
  Divide1 : Product  Inputs=*/
  Gain : Gain  Gain=-1
  Gain1 : Gain  Gain=57.3
  Gain3 : Gain  Gain=180/pi
  Gain4 : Gain  Gain=180/pi
  Gain5 : Gain  Gain=-1
  Mux : Mux  Inputs=3
  Product : Product  Inputs=*/
  Scope{,1..3} (4 alike) : Scope
      Scope settings: ActiveDisplayYMinimum=8.024405871416926  ActiveDisplayYMaximum=8.02525358946757  DataLoggingVariableName=ScopeData9
      Scope1 settings: ActiveDisplayYMinimum=-1  ActiveDisplayYMaximum=1  DataLoggingVariableName=ScopeData10
      Scope2 settings: ActiveDisplayYMinimum=-1  ActiveDisplayYMaximum=1  DataLoggingVariableName=ScopeData11
      Scope3 settings: ActiveDisplayYMinimum=-1  ActiveDisplayYMaximum=1  DataLoggingVariableName=ScopeData12
  Sum : Sum  Inputs=|+-
  Sum1 : Sum  Inputs=|+-
  Sum2 : Sum  Inputs=|+-
  Sum3 : Sum  Inputs=-+|
  Sum4 : Sum  Inputs=-+|
  Sum5 : Sum  Inputs=-+|
  Trigonometric Function : Trigonometry  Operator=atan2
  Trigonometric Function1 : Trigonometry  Operator=asin
  目标运动学模型 : Subsystem
  相对位置 : Scope  NumInputPorts=3
      settings: ActiveDisplayYMinimum=-1300.2467720540753  ActiveDisplayYMaximum=5700.0274191171193  DataLoggingVariableName=ScopeData22
  视线方位角 : Scope
      settings: ActiveDisplayYMinimum=-1  ActiveDisplayYMaximum=1  DataLoggingVariableName=ScopeData14
  视线高低1角 : Scope
      settings: ActiveDisplayYMinimum=-1  ActiveDisplayYMaximum=1  DataLoggingVariableName=ScopeData13
  计算视线角速率 : Subsystem
  距离 : Fcn  Expr=sqrt(u(1)^2+u(2)^2+u(3)^2)
  速度大小 : Fcn  Expr=sqrt(u(1)^2+u(2)^2+u(3)^2)
  俯仰角（弧度） : Outport
  视线高低角速率(弧度) : Outport  Port=2
  视线方位角速率（弧度） : Outport  Port=3
  视线高低角 : Outport  Port=4
  tag scope: R=global
  wires:
  飞行器地面系位置/1 -> Demux1/1
  Demux1/1 -> Sum/2
  Demux1/2 -> Sum1/2
  Demux1/3 -> Sum2/2
  Sum/1 -> Mux/1, 相对位置/1, Trigonometric Function/2, 计算视线角速率/1(rx)  "rx"
  Sum1/1 -> Mux/2, 相对位置/2, Trigonometric Function/1, 计算视线角速率/2(ry)  "ry"
  Sum2/1 -> Gain5/1, 相对位置/3, Mux/3, 计算视线角速率/3(rz)  "rz"
  Mux/1 -> 距离/1
  距离/1 -> 计算视线角速率/4(r), Divide1/2, Scope/1, [R]
  目标运动学模型/4(Vx_t) -> Sum3/1
  目标运动学模型/5(Vy_t) -> Sum4/1
  目标运动学模型/6(Vz_t) -> Sum5/1
  Sum3/1 -> 计算视线角速率/5(Vx)  "vx"
  Sum4/1 -> 计算视线角速率/6(Vy)  "vy"
  Sum5/1 -> 计算视线角速率/7(Vz)  "vz"
  Divide1/1 -> Asin/1
  Trigonometric Function/1 -> Gain4/1
  Gain3/1 -> 视线高低角/1, 视线高低1角/1
  Gain4/1 -> 视线方位角/1
  Asin/1 -> Gain3/1
  Gain5/1 -> Divide1/1
  计算视线角速率/1(视线高低角速率(弧度)) -> Scope1/1, 视线高低角速率(弧度)/1
  计算视线角速率/2(视线方位角速率（弧度）) -> Scope2/1, 视线方位角速率（弧度）/1
  Demux2/2 -> Sum4/2
  Demux2/1 -> Sum3/2
  Product/1 -> Trigonometric Function1/1
  Gain/1 -> Product/1
  Trigonometric Function1/1 -> Gain1/1, 俯仰角（弧度）/1
  Demux2/3 -> Gain/1, Sum5/2
  飞行器地面系速度/1 -> 速度大小/1, Demux2/1
  速度大小/1 -> Product/2
  Gain1/1 -> Scope3/1
  目标运动学模型/1(xt) -> Sum/1
  目标运动学模型/2(yt) -> Sum1/1
  目标运动学模型/3(zt) -> Sum2/1

== system b0307/动力学和运动学/位置积分 ==
  phi : Inport
  theta : Inport  Port=2
  psi : Inport  Port=3
  u : Inport  Port=4
  v : Inport  Port=5
  w : Inport  Port=6
  Demux : Demux  Outputs=3
  Integrator : Integrator
  Integrator1 : Integrator
  Integrator2 : Integrator
  MATLAB Function : MATLAB Function  TreatAsAtomicUnit=on
  Matrix Multiply : Product  Multiplication=Matrix(*)
  Mux : Mux  Inputs=3
  Reshape : Reshape  OutputDimensionality=Column vector (2-D)
  Transpose : matrix_library/Transpose
  x : Outport
  y : Outport  Port=2
  z : Outport  Port=3
  tag scope: V_g=global
  wires:
  Mux/1 -> Reshape/1
  phi/1 -> MATLAB Function/1(phi)
  Matrix Multiply/1 -> [V_g], Demux/1  "地面系速度"
  Demux/1 -> Integrator/1
  Reshape/1 -> Matrix Multiply/2
  Demux/2 -> Integrator1/1
  MATLAB Function/1(R_bg) -> Transpose/1
  Demux/3 -> Integrator2/1
  Integrator/1 -> x/1
  theta/1 -> MATLAB Function/2(theta)
  psi/1 -> MATLAB Function/3(psi)
  u/1 -> Mux/1
  v/1 -> Mux/2
  w/1 -> Mux/3
  Integrator1/1 -> y/1
  Integrator2/1 -> z/1
  Transpose/1 -> Matrix Multiply/1

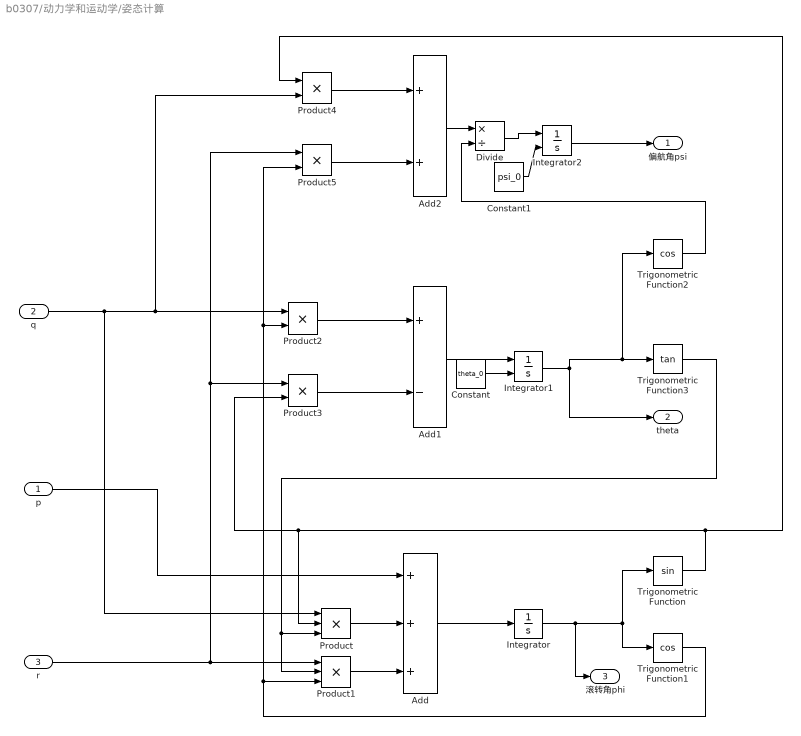
== system b0307/动力学和运动学/姿态计算 ==
  p : Inport
  q : Inport  Port=2
  r : Inport  Port=3
  Add : Sum  Inputs=+++
  Add1 : Sum  Inputs=+-
  Add2 : Sum
  Constant : Constant  Value=theta_0
  Constant1 : Constant  Value=psi_0
  Divide : Product  Inputs=*/
  Integrator : Integrator
  Integrator1 : Integrator  InitialConditionSource=external
  Integrator2 : Integrator  InitialConditionSource=external
  Product : Product  Inputs=3
  Product1 : Product  Inputs=3
  Product{2..5} (4 alike) : Product
  Trigonometric Function : Trigonometry
  Trigonometric Function1 : Trigonometry  Operator=cos
  Trigonometric Function2 : Trigonometry  Operator=cos
  Trigonometric Function3 : Trigonometry  Operator=tan
  偏航角psi : Outport
  theta : Outport  Port=2
  滚转角phi : Outport  Port=3
  wires:
  Add1/1 -> Integrator1/1
  Trigonometric Function1/1 -> Product1/3, Product5/2, Product2/2
  Add2/1 -> Divide/1
  Trigonometric Function2/1 -> Divide/2
  p/1 -> Add/1
  Product2/1 -> Add1/1
  r/1 -> Product5/1, Product3/1, Product1/1
  Integrator1/1 -> Trigonometric Function3/1, Trigonometric Function2/1, theta/1
  Integrator/1 -> 滚转角phi/1, Trigonometric Function1/1, Trigonometric Function/1
  Product4/1 -> Add2/1
  Product/1 -> Add/2
  Trigonometric Function/1 -> Product4/1, Product3/2, Product/2
  Trigonometric Function3/1 -> Product1/2, Product/3
  Divide/1 -> Integrator2/1
  Add/1 -> Integrator/1
  Integrator2/1 -> 偏航角psi/1
  Product5/1 -> Add2/2
  Product1/1 -> Add/3
  q/1 -> Product/1, Product4/2, Product2/1
  Product3/1 -> Add1/2
  Constant/1 -> Integrator1/2
  Constant1/1 -> Integrator2/2

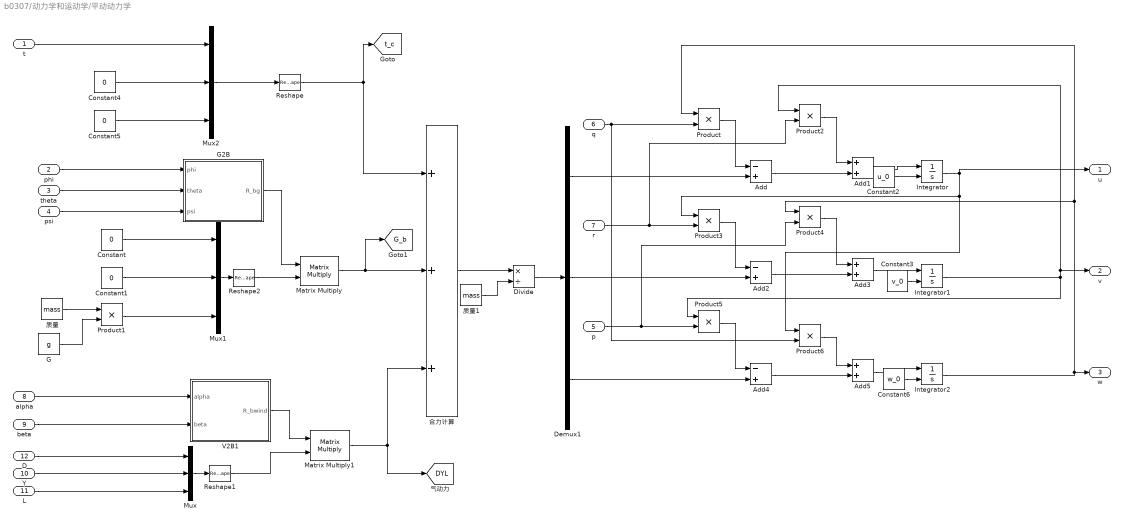
== system b0307/动力学和运动学/平动动力学 ==
  t : Inport
  phi : Inport  Port=2
  theta : Inport  Port=3
  psi : Inport  Port=4
  p : Inport  Port=5
  q : Inport  Port=6
  r : Inport  Port=7
  alpha : Inport  Port=8
  beta : Inport  Port=9
  Y : Inport  Port=10
  L : Inport  Port=11
  D : Inport  Port=12
  Add : Sum  Inputs=-+
  Add1 : Sum
  Add2 : Sum  Inputs=-+
  Add3 : Sum
  Add4 : Sum  Inputs=-+
  Add5 : Sum
  Constant{,1,4..5} (4 alike) : Constant  Value=0
  Constant2 : Constant  Value=u_0
  Constant3 : Constant  Value=v_0
  Constant6 : Constant  Value=w_0
  Demux1 : Demux  Outputs=3
  Divide : Product  Inputs=*/
  G : Constant  Value=g
  G2B : MATLAB Function  TreatAsAtomicUnit=on
  Integrator : Integrator  InitialConditionSource=external
  Integrator1 : Integrator  InitialConditionSource=external
  Integrator2 : Integrator  InitialConditionSource=external
  Matrix Multiply : Product  Multiplication=Matrix(*)
  Matrix Multiply1 : Product  Multiplication=Matrix(*)
  Mux : Mux  Inputs=3
  Mux1 : Mux  Inputs=3
  Mux2 : Mux  Inputs=3
  Product{,1..6} (7 alike) : Product
  Reshape : Reshape  OutputDimensionality=Column vector (2-D)
  Reshape1 : Reshape  OutputDimensionality=Column vector (2-D)
  Reshape2 : Reshape  OutputDimensionality=Column vector (2-D)
  V2B1 : MATLAB Function  TreatAsAtomicUnit=on
  合力计算 : Sum  Inputs=+++
  质量 : Constant  Value=mass
  质量1 : Constant  Value=mass
  u : Outport
  v : Outport  Port=2
  w : Outport  Port=3
  tag scope: DYL=global, G_b=global, t_c=global
  wires:
  Integrator2/1 -> w/1, Product4/1, Product/1
  G/1 -> Product1/2
  Constant5/1 -> Mux2/3
  Add3/1 -> Integrator1/1
  Constant/1 -> Mux1/1
  Constant4/1 -> Mux2/2
  G2B/1(R_bg) -> Matrix Multiply/1
  t/1 -> Mux2/1
  q/1 -> Product6/2, Product/2
  alpha/1 -> V2B1/1(alpha)
  Integrator/1 -> u/1, Product6/1, Product3/1
  Add/1 -> Add1/2
  Y/1 -> Mux/2
  p/1 -> Product5/2, Product4/2
  Mux2/1 -> Reshape/1
  Add5/1 -> Integrator2/1
  Integrator1/1 -> v/1, Product2/1, Product5/1
  V2B1/1(R_bwind) -> Matrix Multiply1/1
  beta/1 -> V2B1/2(beta)
  质量/1 -> Product1/1
  Demux1/2 -> Add2/2
  Mux1/1 -> Reshape2/1
  Reshape2/1 -> Matrix Multiply/2
  Divide/1 -> Demux1/1
  Constant1/1 -> Mux1/2
  Demux1/1 -> Add/2
  Add1/1 -> Integrator/1
  Product5/1 -> Add4/1
  Mux/1 -> Reshape1/1
  Matrix Multiply/1 -> [G_b], 合力计算/2
  质量1/1 -> Divide/2
  Product2/1 -> Add1/1
  Add4/1 -> Add5/2
  Product3/1 -> Add2/1
  Reshape/1 -> [t_c], 合力计算/1
  Demux1/3 -> Add4/2
  Product4/1 -> Add3/1
  L/1 -> Mux/3
  Product/1 -> Add/1
  Add2/1 -> Add3/2
  r/1 -> Product3/2, Product2/2
  Matrix Multiply1/1 -> [DYL], 合力计算/3
  Reshape1/1 -> Matrix Multiply1/2
  合力计算/1 -> Divide/1
  D/1 -> Mux/1
  phi/1 -> G2B/1(phi)
  psi/1 -> G2B/3(psi)
  Product6/1 -> Add5/1
  theta/1 -> G2B/2(theta)
  Constant2/1 -> Integrator/2
  Product1/1 -> Mux1/3
  Constant6/1 -> Integrator2/2
  Constant3/1 -> Integrator1/2

== system b0307/动力学和运动学/触地判断 ==
  z : Inport
  Const1nt1 : Constant  Value=0
  Const1nt2 : Constant
  Gain : Gain  Gain=-1
  Stop Simulation : Stop
  Switch : Switch  Criteria=u2 > Threshold  Threshold=-1  SaturateOnIntegerOverflow=off  InputSameDT=off
  wires:
  z/1 -> Gain/1
  Const1nt2/1 -> Switch/3
  Gain/1 -> Switch/2
  Switch/1 -> Stop Simulation/1
  Const1nt1/1 -> Switch/1

== system b0307/动力学和运动学/转动动力学 ==
  L : Inport
  M : Inport  Port=2
  N : Inport  Port=3
  Add : Sum  Inputs=+-
  Constant : Constant  Value=I
  Constant1 : Constant  Value=I_inv
  Cross Product : matrix_library/Cross Product
  Demux1 : Demux  Outputs=3
  Integrator3 : Integrator
  Integrator4 : Integrator
  Integrator5 : Integrator
  Matrix Multiply1 : Product  Multiplication=Matrix(*)
  Mux : Mux  Inputs=3
  Mux2 : Mux  Inputs=3
  Product2 : Product  Multiplication=Matrix(*)
  p : Outport  VectorParamsAs1DForOutWhenUnconnected=off
  q : Outport  Port=2  VectorParamsAs1DForOutWhenUnconnected=off
  r : Outport  Port=3  VectorParamsAs1DForOutWhenUnconnected=off
  wires:
  N/1 -> Mux/3
  L/1 -> Mux/1
  M/1 -> Mux/2
  Mux/1 -> Add/1
  Demux1/3 -> Integrator4/1
  Demux1/1 -> Integrator3/1
  Demux1/2 -> Integrator5/1
  Integrator4/1 -> Mux2/3, r/1
  Integrator5/1 -> Mux2/2, q/1
  Integrator3/1 -> Mux2/1, p/1
  Matrix Multiply1/1 -> Demux1/1
  Constant1/1 -> Matrix Multiply1/1
  Add/1 -> Matrix Multiply1/2
  Constant/1 -> Product2/1
  Mux2/1 -> Cross Product/1, Product2/2
  Product2/1 -> Cross Product/2
  Cross Product/1 -> Add/2

== system b0307/气动力和气动力矩/气动力 ==
  q_p : Inport
  beta : Inport  Port=2
  alpha : Inport  Port=3
  delta_l : Inport  Port=4
  delta_r : Inport  Port=5
  侧力 : Subsystem
  升力 : Subsystem
  阻力 : Subsystem
  阻力D : Outport
  侧力Y : Outport  Port=2
  升力L : Outport  Port=3
  wires:
  alpha/1 -> 阻力/3(alpha1), 侧力/3(alpha1), 升力/3(alpha)
  q_p/1 -> 阻力/1(q_p1), 侧力/1(q_p1), 升力/1(q_p)
  升力/1(升力L) -> 升力L/1
  beta/1 -> 阻力/2(beta1), 侧力/2(beta1), 升力/2(beta)
  阻力/1(阻力L) -> 阻力D/1
  侧力/1(侧力Y) -> 侧力Y/1
  delta_l/1 -> 阻力/4(delta_l), 侧力/4(delta_l), 升力/4(delta_l)
  delta_r/1 -> 阻力/5(delta_r), 侧力/5(delta_r), 升力/5(delta_r)

== system b0307/气动力和气动力矩/气动力矩 ==
  q_p : Inport
  beta : Inport  Port=2
  alpha : Inport  Port=3
  delta_l : Inport  Port=4
  delta_r : Inport  Port=5
  俯仰力矩 : Subsystem
  偏航力矩 : Subsystem
  滚转力矩 : Subsystem
  滚转力矩l : Outport
  俯仰力矩m : Outport  Port=2
  偏航力矩n : Outport  Port=3
  wires:
  alpha/1 -> 滚转力矩/3(alpha1), 俯仰力矩/3(alpha1), 偏航力矩/3(alpha)
  q_p/1 -> 滚转力矩/1(q_p1), 俯仰力矩/1(q_p1), 偏航力矩/1(q_p)
  偏航力矩/1(偏航力矩) -> 偏航力矩n/1
  beta/1 -> 滚转力矩/2(beta1), 俯仰力矩/2(beta1), 偏航力矩/2(beta)
  滚转力矩/1(滚转力矩) -> 滚转力矩l/1
  俯仰力矩/1(俯仰力矩) -> 俯仰力矩m/1
  delta_r/1 -> 滚转力矩/5(delta_r), 俯仰力矩/5(delta_r), 偏航力矩/5(delta_r)
  delta_l/1 -> 滚转力矩/4(delta_l), 俯仰力矩/4(delta_l), 偏航力矩/4(delta_l)

== system b0307/俯仰过载控制器和滚转姿态控制器/俯仰过载控制器/计算过载 ==
  Add : Sum
  Demux : Demux  Outputs=3
  Product10 : Product  Inputs=*/
  nz : Outport
  wires:
  [t_c] -> Add/1
  Product10/1 -> Demux/1
  [DYL] -> Add/2
  Demux/3 -> nz/1
  Add/1 -> Product10/1
  [G_b] -> Product10/2

== system b0307/制导系统/制导系统/BTT ==
  法向过载指令 : Inport
  横向过载指令 : Inport  Port=2
  Abs1 : Abs  SaturateOnIntegerOverflow=off
  Abs2 : Abs  SaturateOnIntegerOverflow=off
  Constant1 : Constant  Value=30
  Constant2 : Constant  Value=3
  Gain11 : Gain  Gain=180/pi
  MinMax : MinMax  Inputs=2
  MinMax1 : MinMax  Inputs=2
  Product1 : Product
  Product2 : Product
  Scope{1..4} (4 alike) : Scope
      Scope1 settings: ActiveDisplayYMinimum=-15.509988320844872  ActiveDisplayYMaximum=15.500965322115452  DataLoggingVariableName=ScopeData2
      Scope2 settings: ActiveDisplayYMinimum=-2.5274340870033787  ActiveDisplayYMaximum=0.98557269309004292  DataLoggingVariableName=ScopeData19
      Scope3 settings: ActiveDisplayYMinimum=-0.37470864763943429  ActiveDisplayYMaximum=0.36718860571372275  DataLoggingVariableName=ScopeData20
      Scope4 settings: ActiveDisplayYMinimum=-2.526030820071004  ActiveDisplayYMaximum=0.98540779257165645  DataLoggingVariableName=ScopeData28
  Sign : Signum
  Sign1 : Signum
  btt : MATLAB Function  TreatAsAtomicUnit=on
  体轴系法向过载 : Outport
  滚转角指令 : Outport  Port=2
  wires:
  Constant2/1 -> MinMax/2
  横向过载指令/1 -> Scope3/1, btt/2(ny_c)
  btt/2(phi_c) -> Gain11/1
  btt/1(nz_b) -> Sign/1, Abs1/1
  Abs1/1 -> MinMax/1
  Product2/1 -> 体轴系法向过载/1, Scope4/1
  Sign/1 -> Product2/1
  MinMax/1 -> Product2/2
  法向过载指令/1 -> Scope2/1, btt/1(nz_c)
  Gain11/1 -> Abs2/1, Sign1/1
  Sign1/1 -> Product1/1
  Abs2/1 -> MinMax1/1
  MinMax1/1 -> Product1/2
  Constant1/1 -> MinMax1/2
  Product1/1 -> 滚转角指令/1, Scope1/1

== system b0307/制导系统/制导系统/巡航段制导 ==
  dy1 : Inport
  dy_dot : Inport  Port=2
  航向制导回路 : Subsystem
  高度控制回路 : Subsystem
  Nzc : Outport
  Nyc : Outport  Port=2
  wires:
  [V_g] -> 高度控制回路/1(速度)
  高度控制回路/1(Nzc) -> Nzc/1
  航向制导回路/1(Nyc) -> Nyc/1
  dy_dot/1 -> 航向制导回路/1(速度)
  dy1/1 -> 航向制导回路/2(侧偏)

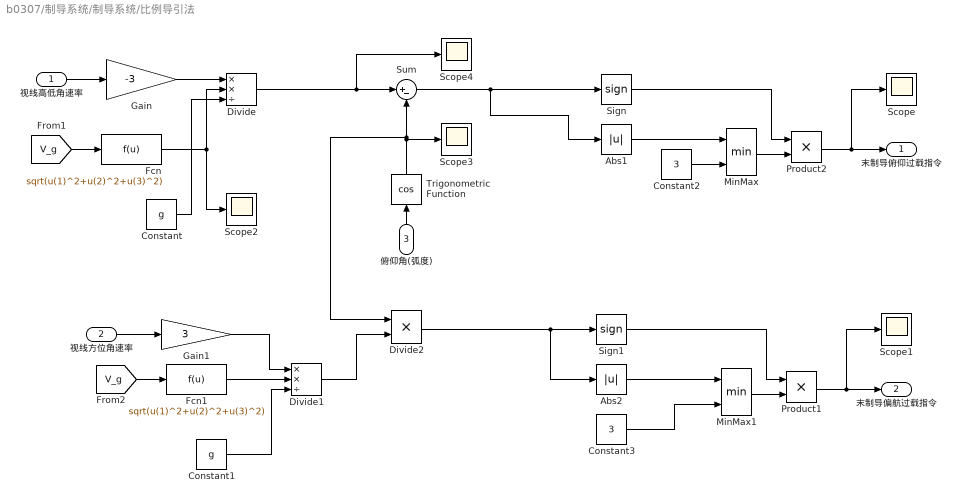
== system b0307/制导系统/制导系统/比例导引法 ==
  视线高低角速率 : Inport
  视线方位角速率 : Inport  Port=2
  俯仰角(弧度) : Inport  Port=3
  Abs1 : Abs  SaturateOnIntegerOverflow=off
  Abs2 : Abs  SaturateOnIntegerOverflow=off
  Constant : Constant  Value=g
  Constant1 : Constant  Value=g
  Constant2 : Constant  Value=3
  Constant3 : Constant  Value=3
  Divide : Product  Inputs=**/
  Divide1 : Product  Inputs=**/
  Divide2 : Product  Inputs=**
  Fcn : Fcn  Expr=sqrt(u(1)^2+u(2)^2+u(3)^2)
  Fcn1 : Fcn  Expr=sqrt(u(1)^2+u(2)^2+u(3)^2)
  Gain : Gain  Gain=-3
  Gain1 : Gain  Gain=3
  MinMax : MinMax  Inputs=2
  MinMax1 : MinMax  Inputs=2
  Product1 : Product
  Product2 : Product
  Scope{,1..4} (5 alike) : Scope
      Scope settings: ActiveDisplayYMinimum=-1  ActiveDisplayYMaximum=1  DataLoggingVariableName=ScopeData15
      Scope1 settings: ActiveDisplayYMinimum=-0.061498666278822167  ActiveDisplayYMaximum=0.144706541855943  DataLoggingVariableName=ScopeData16
      Scope2 settings: ActiveDisplayYMinimum=-1  ActiveDisplayYMaximum=1  DataLoggingVariableName=ScopeData17
      Scope3 settings: ActiveDisplayYMinimum=-1  ActiveDisplayYMaximum=1  DataLoggingVariableName=ScopeData21
      Scope4 settings: ActiveDisplayYMinimum=-0.48030962065940375  ActiveDisplayYMaximum=1.1590901854759237  DataLoggingVariableName=ScopeData23
  Sign : Signum
  Sign1 : Signum
  Sum : Sum  Inputs=|+-
  Trigonometric Function : Trigonometry  Operator=cos
  末制导俯仰过载指令 : Outport
  末制导偏航过载指令 : Outport  Port=2
  wires:
  [V_g] -> Fcn/1
  Constant/1 -> Divide/3
  Constant1/1 -> Divide1/3
  Gain1/1 -> Divide1/1
  视线方位角速率/1 -> Gain1/1
  [V_g] -> Fcn1/1
  俯仰角(弧度)/1 -> Trigonometric Function/1
  Product2/1 -> Scope/1, 末制导俯仰过载指令/1
  Sign/1 -> Product2/1
  Constant2/1 -> MinMax/2
  Abs1/1 -> MinMax/1
  MinMax/1 -> Product2/2
  MinMax1/1 -> Product1/2
  Product1/1 -> 末制导偏航过载指令/1, Scope1/1
  Sign1/1 -> Product1/1
  Abs2/1 -> MinMax1/1
  Constant3/1 -> MinMax1/2
  Divide2/1 -> Abs2/1, Sign1/1
  Fcn/1 -> Scope2/1, Divide/2
  Fcn1/1 -> Divide1/2
  Trigonometric Function/1 -> Sum/2, Divide2/1, Scope3/1
  Divide1/1 -> Divide2/2
  Gain/1 -> Divide/1
  Sum/1 -> Abs1/1, Sign/1
  视线高低角速率/1 -> Gain/1
  Divide/1 -> Scope4/1, Sum/1

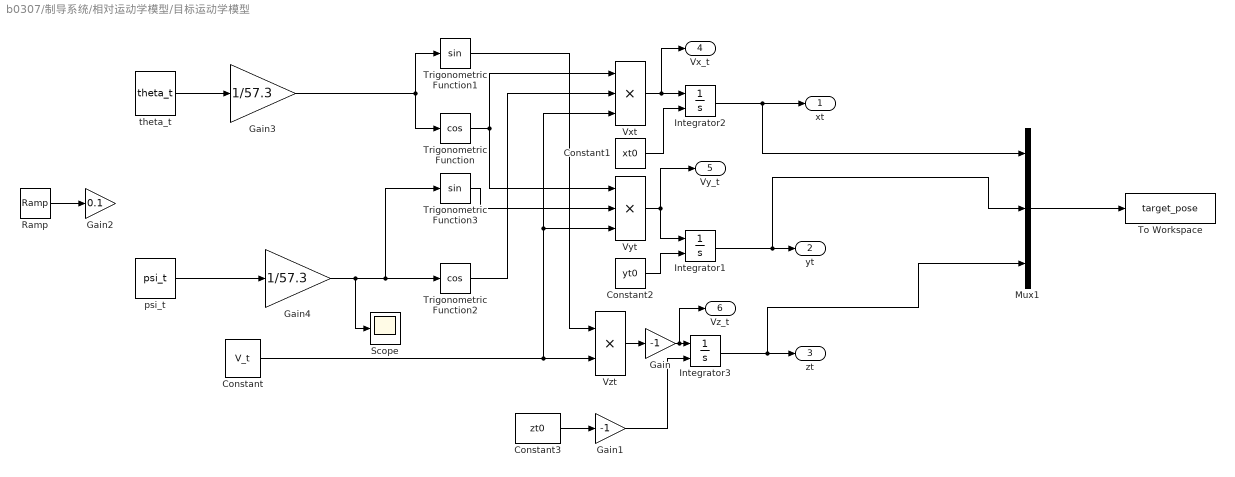
== system b0307/制导系统/相对运动学模型/目标运动学模型 ==
  Constant : Constant  Value=V_t
  Constant1 : Constant  Value=xt0
  Constant2 : Constant  Value=yt0
  Constant3 : Constant  Value=zt0
  Gain : Gain  Gain=-1
  Gain1 : Gain  Gain=-1
  Gain2 : Gain  Gain=0.1
  Gain3 : Gain  Gain=1/57.3
  Gain4 : Gain  Gain=1/57.3
  Integrator1 : Integrator  InitialConditionSource=external
  Integrator2 : Integrator  InitialConditionSource=external
  Integrator3 : Integrator  InitialConditionSource=external
  Mux1 : Mux  Inputs=3
  Ramp : simulink/Sources/Ramp  slope=15  start=0  InitialOutput=0
  Scope : Scope
      settings: ActiveDisplayYMinimum=-1  ActiveDisplayYMaximum=1  DataLoggingVariableName=ScopeData18
  To Workspace : ToWorkspace  VariableName=target_pose  SaveFormat=Timeseries  SampleTime=-1
  Trigonometric Function : Trigonometry  Operator=cos
  Trigonometric Function1 : Trigonometry
  Trigonometric Function2 : Trigonometry  Operator=cos
  Trigonometric Function3 : Trigonometry
  Vxt : Product  Inputs=3
  Vyt : Product  Inputs=3
  Vzt : Product
  psi_t : Constant  Value=psi_t
  theta_t : Constant  Value=theta_t
  xt : Outport
  yt : Outport  Port=2
  zt : Outport  Port=3
  Vx_t : Outport  Port=4
  Vy_t : Outport  Port=5
  Vz_t : Outport  Port=6
  wires:
  theta_t/1 -> Gain3/1
  Constant/1 -> Vyt/3, Vxt/3, Vzt/2
  Trigonometric Function2/1 -> Vxt/2
  Trigonometric Function/1 -> Vyt/1, Vxt/1
  Trigonometric Function3/1 -> Vyt/2
  Trigonometric Function1/1 -> Vzt/1
  Vxt/1 -> Vx_t/1, Integrator2/1
  Vyt/1 -> Vy_t/1, Integrator1/1
  Vzt/1 -> Gain/1
  Constant1/1 -> Integrator2/2
  Constant2/1 -> Integrator1/2
  Constant3/1 -> Gain1/1
  Gain/1 -> Vz_t/1, Integrator3/1
  Gain1/1 -> Integrator3/2
  Gain3/1 -> Trigonometric Function/1, Trigonometric Function1/1
  Integrator3/1 -> Mux1/3, zt/1
  Mux1/1 -> To Workspace/1
  Integrator2/1 -> Mux1/1, xt/1
  Integrator1/1 -> Mux1/2, yt/1
  psi_t/1 -> Gain4/1
  Ramp/1 -> Gain2/1
  Gain4/1 -> Scope/1, Trigonometric Function2/1, Trigonometric Function3/1

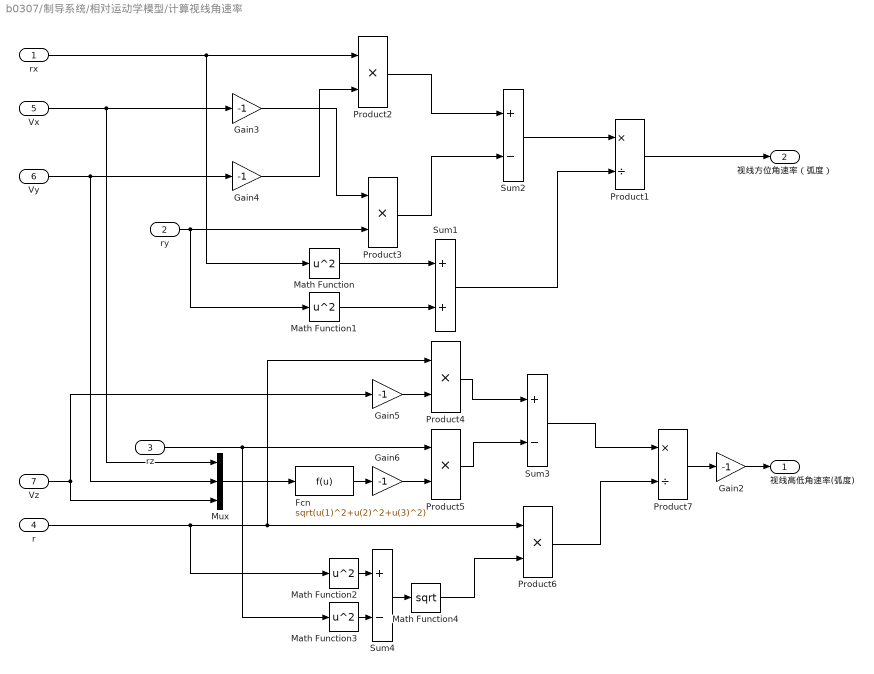
== system b0307/制导系统/相对运动学模型/计算视线角速率 ==
  rx : Inport
  ry : Inport  Port=2
  rz : Inport  Port=3
  r : Inport  Port=4
  Vx : Inport  Port=5
  Vy : Inport  Port=6
  Vz : Inport  Port=7
  Fcn : Fcn  Expr=sqrt(u(1)^2+u(2)^2+u(3)^2)
  Gain{2..6} (5 alike) : Gain  Gain=-1
  Math Function{,1..3} (4 alike) : Math  Operator=square  SignedPower=on
  Math Function4 : Math  Operator=sqrt  SignedPower=on
  Mux : Mux  Inputs=3
  Product1 : Product  Inputs=*/  RndMeth=Zero
  Product{2..6} (5 alike) : Product  RndMeth=Zero
  Product7 : Product  Inputs=*/  RndMeth=Zero
  Sum1 : Sum  Inputs=2
  Sum2 : Sum  Inputs=+-
  Sum3 : Sum  Inputs=+-
  Sum4 : Sum  Inputs=+-
  视线高低角速率(弧度) : Outport  VectorParamsAs1DForOutWhenUnconnected=off
  视线方位角速率（弧度） : Outport  Port=2  VectorParamsAs1DForOutWhenUnconnected=off
  wires:
  rz/1 -> Product5/1, Math Function3/1
  Gain4/1 -> Product2/2
  Gain3/1 -> Product3/1
  Product2/1 -> Sum2/1
  Product3/1 -> Sum2/2
  Sum2/1 -> Product1/1
  Math Function/1 -> Sum1/1
  Math Function1/1 -> Sum1/2
  Sum1/1 -> Product1/2
  Gain5/1 -> Product4/2
  Product4/1 -> Sum3/1
  Product5/1 -> Sum3/2
  Math Function2/1 -> Sum4/1
  Math Function3/1 -> Sum4/2
  Sum4/1 -> Math Function4/1
  Math Function4/1 -> Product6/2
  Product6/1 -> Product7/2
  Product7/1 -> Gain2/1
  Product1/1 -> 视线方位角速率（弧度）/1
  Sum3/1 -> Product7/1
  Fcn/1 -> Gain6/1
  r/1 -> Product6/1, Product4/1, Math Function2/1
  ry/1 -> Math Function1/1, Product3/2
  Vx/1 -> Gain3/1, Mux/1
  Vy/1 -> Gain4/1, Mux/2
  Vz/1 -> Gain5/1, Mux/3
  Mux/1 -> Fcn/1
  Gain6/1 -> Product5/2
  rx/1 -> Product2/1, Math Function/1
  Gain2/1 -> 视线高低角速率(弧度)/1
